simulink model "HAE"  (R2018a)
settings: Solver=ode4  StartTime=0  StopTime=2  MaxStep=1e-4  RelTol=1e-3
InitFcn:
  | close
  | clear
  | clc
  | Sc=128
  | f=60;
  | T=1/f;
  | Ts=1/(f*Sc);
  | Vr=6500
  | V_v=[1    0.4    1          0.6       1       0.6       1       0.75   0.95]
  | T_v=[0   20/f  70/f    200/f   300/f     330/f   400/f   500/f  10]
  | S_time=60/f*20.5
  | V_R=3;
  | Tf=3
  | T_lc=3
  | set_param('HAE/EMISOR-RECEPTOR/TCP_IP_RX1/ESCRITURA', 'Value','0')
  | set_param('HAE/EMISOR-RECEPTOR/TCP_IP_RX1/RETARDO', 'Value','0')
  | run script_client_1_inicio2.m
undefined symbols (not defined in the file or in its folder): D11, Delta, DiscIntNeverNeededParam, Int, Ip1
libraries: powerlib x68, simulink x12, powerlib_meascontrol x6, libreria_comunicaciones_cliente2 x2, libreria_medidores2 x1
(part 3 of 5)

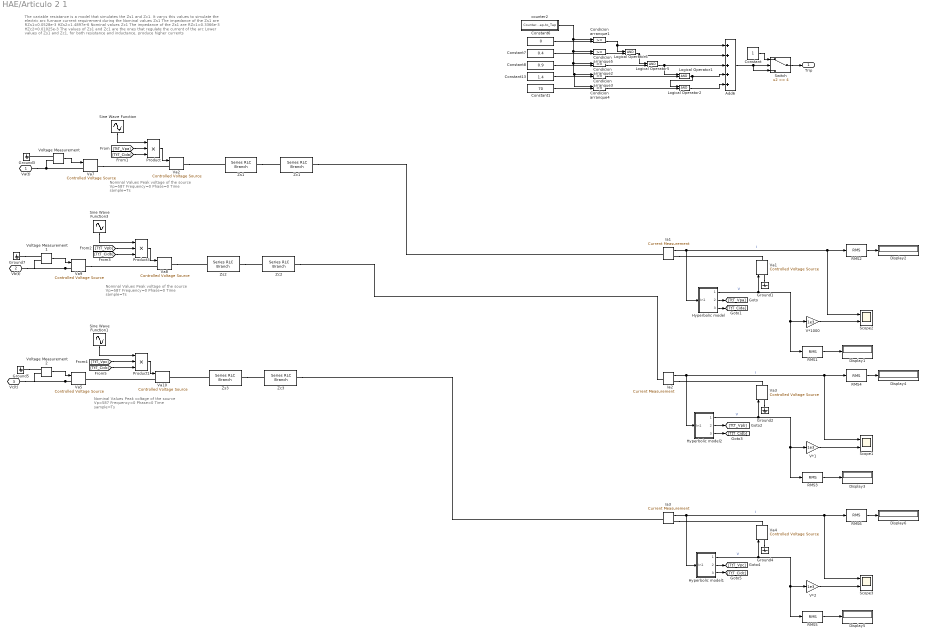
== system HAE/Articulo 2 1 ==
  note: The variable resistance is a model that simulates the Zs1 and Zc1. It varys this values to simulate the electric arc furnace current requirement during the
      |
      | Nominal values  Zs1
      | The impedance of the Zs1 are
      | RZs1=0.0528e-3
      | HZs2=1.4897e-6
      |
      | Nominal values Zc1
      | The impedance of the Zs1 are
      | RZc1=0.3366e-3
      | HZc2=0.01025e-3
      |
      |
      | The values of Zs1 and Zc1 are the ones that regulate the current of the arc
      |
      | Lower values of Zs1 and Zc1, for both resistance and inductance, produce higher currents
  note: Nominal Values
      |
      | Peak voltage of the source Vp=587
      | Frequency=0
      | Phase=0
      | Time sample=Ts
  note: Nominal Values
      |
      | Peak voltage of the source Vp=587
      | Frequency=0
      | Phase=0
      | Time sample=Ts
  note: Nominal Values
      |
      | Peak voltage of the source Vp=587
      | Frequency=0
      | Phase=0
      | Time sample=Ts
  Add6 : Sum  Inputs=+++++
  Condicion arranque{1..5} (5 alike) : RelationalOperator  OutDataTypeStr=boolean  RndMeth=Nearest
  Constant : Constant
  Constant1 : Constant  Value=70  VectorParams1D=off  SampleTime=Ts
  Constant13 : Constant  Value=1.4  VectorParams1D=off  SampleTime=Ts
  Constant6 : Constant  Value=0  VectorParams1D=off  SampleTime=Ts
  Constant7 : Constant  Value=0.4  VectorParams1D=off  SampleTime=Ts
  Constant8 : Constant  Value=0.9  VectorParams1D=off  SampleTime=Ts
  Display{1..6} (6 alike) : Display
  Ground{1..5,7} (6 alike) : powerlib/Elements/Ground  LConnTagsString=a
  Hyperbolic model : Subsystem
  Hyperbolic model1 : Subsystem
  Hyperbolic model2 : Subsystem
  Ia1 : powerlib/Measurements/Current Measurement  PhasorSimulation=off  OutputType=Complex  PSBequivalent=0
  Ia2 : powerlib/Measurements/Current Measurement  PhasorSimulation=off  OutputType=Complex  PSBequivalent=0
  Ia3 : powerlib/Measurements/Current Measurement  PhasorSimulation=off  OutputType=Complex  PSBequivalent=0
  Logical Operator{1..2,5..6} (4 alike) : Logic  AllPortsSameDT=off  OutDataTypeStr=boolean
  Product : Product  Inputs=3
  Product1 : Product  Inputs=3
  Product3 : Product  Inputs=3
  RMS{1..6} (6 alike) : powerlib_meascontrol/Measurements/RMS  TrueRMS=on  Freq=60  RMSInit=120  Ts=Ts
  Scope1 : Scope  NumInputPorts=2
  Scope2 : Scope  NumInputPorts=2
  Scope3 : Scope  NumInputPorts=2
  Sine Wave Function : Sin  Amplitude=Vp  Frequency=60*2*pi  Phase=pi/8  SampleTime=Ts
  Sine Wave Function1 : Sin  Amplitude=Vp  Frequency=60*2*pi  Phase=-2*pi/3  SampleTime=Ts
  Sine Wave Function3 : Sin  Amplitude=Vp  Frequency=60*2*pi  Phase=2*pi/3  SampleTime=Ts
  Switch : Switch  Threshold=4
  V*1 : Gain  Gain=1e3
  V*1000 : Gain  Gain=1e3
  V*2 : Gain  Gain=1e3
  Va1 : powerlib/Electrical Sources/Controlled Voltage Source  Initialize=on  Source_Type=AC  Amplitude=0  Phase=0  Frequency=0  Measurements=None
  Va{2,5,7..10} (6 alike) : powerlib/Electrical Sources/Controlled Voltage Source  Initialize=on  Source_Type=AC  Amplitude=570  Phase=0  Frequency=60  Measurements=None
  Va3 : powerlib/Electrical Sources/Controlled Voltage Source  Initialize=on  Source_Type=AC  Amplitude=0  Phase=0  Frequency=0  Measurements=None
  Va4 : powerlib/Electrical Sources/Controlled Voltage Source  Initialize=on  Source_Type=AC  Amplitude=0  Phase=0  Frequency=0  Measurements=None
  Voltage Measurement : powerlib/Measurements/Voltage Measurement  PhasorSimulation=off  OutputType=Complex  PSBequivalent=0
  Voltage Measurement1 : powerlib/Measurements/Voltage Measurement  PhasorSimulation=off  OutputType=Complex  PSBequivalent=0
  Voltage Measurement2 : powerlib/Measurements/Voltage Measurement  PhasorSimulation=off  OutputType=Complex  PSBequivalent=0
  Zc1 : powerlib/Elements/Series RLC Branch  LConnTagsString=__new0  RConnTagsString=__new0  BranchType=RL  Resistance=RZc1  Inductance=HZc1  SetiL0=off  InitialCurrent=0  Capacitance=0  Setx0=off  InitialVoltage=0  Measurements=None
  Zc2 : powerlib/Elements/Series RLC Branch  LConnTagsString=__new0  RConnTagsString=__new0  BranchType=RL  Resistance=RZc1  Inductance=HZc1  SetiL0=off  InitialCurrent=0  Capacitance=0  Setx0=off  InitialVoltage=0  Measurements=None
  Zc3 : powerlib/Elements/Series RLC Branch  LConnTagsString=__new0  RConnTagsString=__new0  BranchType=RL  Resistance=RZc1  Inductance=HZc1  SetiL0=off  InitialCurrent=0  Capacitance=0  Setx0=off  InitialVoltage=0  Measurements=None
  Zs1 : powerlib/Elements/Series RLC Branch  LConnTagsString=__new0  RConnTagsString=__new0  BranchType=RL  Resistance=RZs1  Inductance=HZs1  SetiL0=off  InitialCurrent=20e3  Capacitance=0  Setx0=off  InitialVoltage=0  Measurements=None
  Zs2 : powerlib/Elements/Series RLC Branch  LConnTagsString=__new0  RConnTagsString=__new0  BranchType=RL  Resistance=RZs1  Inductance=HZs1  SetiL0=off  InitialCurrent=20e3  Capacitance=0  Setx0=off  InitialVoltage=0  Measurements=None
  Zs3 : powerlib/Elements/Series RLC Branch  LConnTagsString=__new0  RConnTagsString=__new0  BranchType=RL  Resistance=RZs1  Inductance=HZs1  SetiL0=off  InitialCurrent=20e3  Capacitance=0  Setx0=off  InitialVoltage=0  Measurements=None
  counter2 : Subsystem
  Va(t) : PMIOPort  Side=Left
  Vb(t) : PMIOPort  Port=2  Side=Left
  Vc(t) : PMIOPort  Port=3  Side=Left
  Trip : Outport
  wires:
  [TtT_Cida] -> Product/3
  Hyperbolic model/3(TtT_Cid) -> [TtT_Cida]
  [TtT_Vpa] -> Product/2
  Hyperbolic model/2(TtT_Vp) -> [TtT_Vpa]
  Product/1 -> Va2/1
  Sine Wave Function/1 -> Product/1
  Ia1/1 -> RMS2/1, Scope2/1, Hyperbolic model/1(In1)  "I"
  RMS2/1 -> Display2/1
  RMS1/1 -> Display1/1
  V*1000/1 -> Scope2/2
  Hyperbolic model/1(Varc) -> V*1000/1, RMS1/1, Va1/1  "V"
  Hyperbolic model2/3(TtT_Cid) -> [TtT_Cidb]
  Hyperbolic model2/2(TtT_Vp) -> [TtT_Vpb]
  Ia2/1 -> Hyperbolic model2/1(In1), RMS4/1, Scope1/1  "I"
  RMS4/1 -> Display4/1
  RMS3/1 -> Display3/1
  V*1/1 -> Scope1/2
  Hyperbolic model2/1(Varc) -> V*1/1, RMS3/1, Va3/1  "V"
  Hyperbolic model1/3(TtT_Cid) -> [TtT_Cidc]
  Hyperbolic model1/2(TtT_Vp) -> [TtT_Vpc]
  Ia3/1 -> Hyperbolic model1/1(In1), RMS6/1, Scope3/1  "I"
  RMS6/1 -> Display6/1
  RMS5/1 -> Display5/1
  V*2/1 -> Scope3/2
  Hyperbolic model1/1(Varc) -> V*2/1, RMS5/1, Va4/1  "V"
  Voltage Measurement/1 -> Va7/1
  Product3/1 -> Va8/1
  Sine Wave Function3/1 -> Product3/1
  Voltage Measurement1/1 -> Va9/1
  [TtT_Vpb] -> Product3/2
  [TtT_Cidb] -> Product3/3
  Product1/1 -> Va10/1
  Sine Wave Function1/1 -> Product1/1
  Voltage Measurement2/1 -> Va5/1
  [TtT_Vpc] -> Product1/2
  [TtT_Cidc] -> Product1/3
  Add6/1 -> Switch/3, Switch/2
  Constant13/1 -> Condicion arranque3/2
  Condicion arranque1/1 -> Logical Operator6/1, Add6/1
  Condicion arranque3/1 -> Logical Operator1/2
  Logical Operator6/1 -> Add6/2, Logical Operator5/1
  Condicion arranque5/1 -> Logical Operator6/2
  Condicion arranque2/1 -> Logical Operator5/2
  Logical Operator5/1 -> Logical Operator1/1, Add6/3
  Constant6/1 -> Condicion arranque1/2
  Constant8/1 -> Condicion arranque2/2
  Constant7/1 -> Condicion arranque5/2
  Logical Operator1/1 -> Logical Operator2/1, Add6/4
  counter2/1(Counter Tap-to_Tap) -> Condicion arranque5/1, Condicion arranque4/1, Condicion arranque3/1, Condicion arranque2/1, Condicion arranque1/1
  Logical Operator2/1 -> Add6/5
  Condicion arranque4/1 -> Logical Operator2/2
  Constant1/1 -> Condicion arranque4/2
  Switch/1 -> Trip/1
  Constant/1 -> Switch/1
  connections:
  Zc3/RConn1 -- Ia3/LConn1
  Zc2/RConn1 -- Ia2/LConn1
  Zc1/RConn1 -- Ia1/LConn1
  Va1/LConn1 -- Ground1/LConn1
  Zs1/RConn1 -- Zc1/LConn1
  Ia1/RConn1 -- Va1/RConn1
  Va8/RConn1 -- Zs2/LConn1
  Va3/LConn1 -- Ground2/LConn1
  Zs2/RConn1 -- Zc2/LConn1
  Ia2/RConn1 -- Va3/RConn1
  Va4/LConn1 -- Ground4/LConn1
  Zs3/RConn1 -- Zc3/LConn1
  Ia3/RConn1 -- Va4/RConn1
  Va2/RConn1 -- Zs1/LConn1
  Va(t)/RConn1 -- Voltage Measurement/LConn2 -- Va7/LConn1
  Va7/RConn1 -- Va2/LConn1
  Voltage Measurement/LConn1 -- Ground3/LConn1
  Va9/LConn1 -- Vb(t)/RConn1 -- Voltage Measurement1/LConn2
  Va9/RConn1 -- Va8/LConn1
  Ground7/LConn1 -- Voltage Measurement1/LConn1
  Va5/LConn1 -- Vc(t)/RConn1 -- Voltage Measurement2/LConn2
  Ground5/LConn1 -- Voltage Measurement2/LConn1
  Va10/LConn1 -- Va5/RConn1
  Zs3/LConn1 -- Va10/RConn1

== system HAE/EMISOR-RECEPTOR ==
  note: Transmisión de datos
  note: Recepción de datos
  In1 : Inport
  Data Type Conversion : DataTypeConversion  OutDataTypeStr=double
  Scope3 : Scope
  TCP_IP_RX1 : libreria_comunicaciones_cliente2/TCP_IP_RX1  SystemSampleTime=-1
      link override ESCRITURA: Value=client_1.dato_lectura
      link override RETARDO: Value=e
  TCP_IP_TX1 : libreria_comunicaciones_cliente2/TCP_IP_TX1  SystemSampleTime=-1
  Out1 : Outport
  wires:
  TCP_IP_RX1/1 -> Out1/1
  Data Type Conversion/1 -> TCP_IP_TX1/1
  In1/1 -> Scope3/1, Data Type Conversion/1

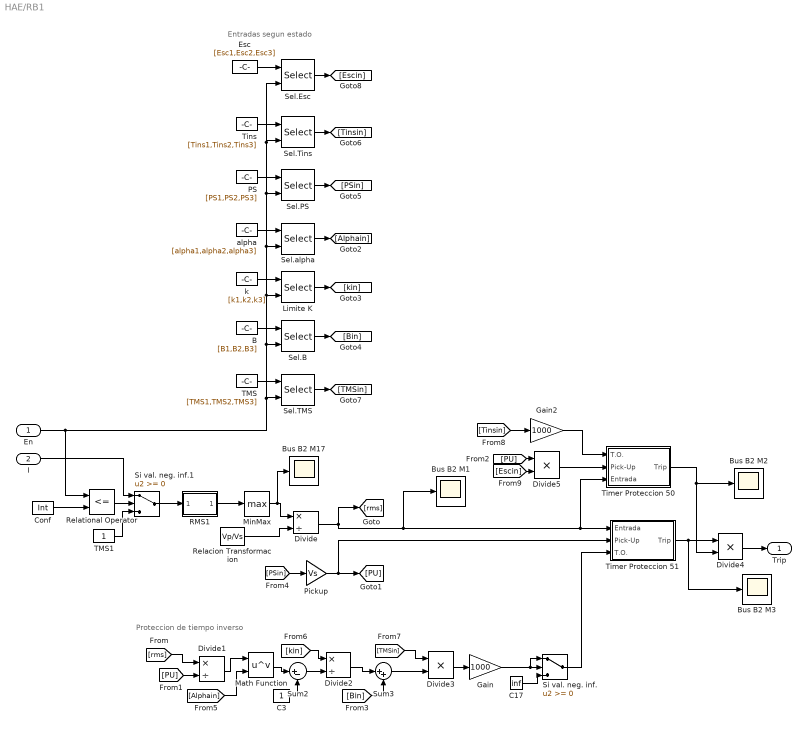
== system HAE/RB1 ==
  note: Proteccion de tiempo inverso
  note: Entradas segun estado
  En : Inport
  I : Inport  Port=2
  B : Constant  Value=[B1,B2,B3]
  Bus B2 M{1..3,17} (4 alike) : Scope
  C17 : Constant  Value=inf
  C3 : Constant
  Conf : Constant  Value=Int
  Divide : Product  Inputs=*/
  Divide1 : Product  Inputs=*/
  Divide2 : Product  Inputs=*/
  Divide3 : Product  Inputs=**
  Divide4 : Product  Inputs=**
  Divide5 : Product  Inputs=**
  Esc : Constant  Value=[Esc1,Esc2,Esc3]
  Gain : Gain  Gain=1000
  Gain2 : Gain  Gain=1000
  Limite K : Selector  InputPortWidth=3  IndexOptions=Index vector (port)  Indices=[1 2 3]  OutputSizes=1
  Math Function : Math  Operator=pow  SaturateOnIntegerOverflow=on
  MinMax : MinMax  Function=max
  PS : Constant  Value=[PS1,PS2,PS3]
  Pickup : Gain  Gain=Vs
  RMS1 : Subsystem
  Relacion Transformacion : Constant  Value=Vp/Vs
  Relational Operator : RelationalOperator  Operator=<=  OutDataTypeStr=boolean  RndMeth=Simplest
  Sel.B : Selector  InputPortWidth=3  IndexOptions=Index vector (port)  Indices=[1 2 3]  OutputSizes=1
  Sel.Esc : Selector  InputPortWidth=3  IndexOptions=Index vector (port)  Indices=[1 2 3]  OutputSizes=1
  Sel.PS : Selector  InputPortWidth=3  IndexOptions=Index vector (port)  Indices=[1 2 3]  OutputSizes=1
  Sel.TMS : Selector  InputPortWidth=3  IndexOptions=Index vector (port)  Indices=[1 2 3]  OutputSizes=1
  Sel.Tins : Selector  InputPortWidth=3  IndexOptions=Index vector (port)  Indices=[1 2 3]  OutputSizes=1
  Sel.alpha : Selector  InputPortWidth=3  IndexOptions=Index vector (port)  Indices=[1 2 3]  OutputSizes=1
  Si val. neg. inf. : Switch
  Si val. neg. inf.1 : Switch
  Sum2 : Sum  Inputs=|+-
  Sum3 : Sum  Inputs=|++
  TMS : Constant  Value=[TMS1,TMS2,TMS3]
  TMS1 : Constant
  Timer Proteccion 50 : Subsystem
  Timer Proteccion 51 : Subsystem
  Tins : Constant  Value=[Tins1,Tins2,Tins3]
  alpha : Constant  Value=[alpha1,alpha2,alpha3]
  k : Constant  Value=[k1,k2,k3]
  Trip : Outport
  wires:
  En/1 -> Relational Operator/1, Sel.TMS/2, Sel.B/2, Limite K/2, Sel.alpha/2, Sel.PS/2, Sel.Tins/2, Sel.Esc/2
  Divide4/1 -> Trip/1
  Tins/1 -> Sel.Tins/1
  [Escin] -> Divide5/2
  Sel.Esc/1 -> [Escin]
  C17/1 -> Si val. neg. inf./3
  Esc/1 -> Sel.Esc/1
  Math Function/1 -> Sum2/1
  [kin] -> Divide2/1
  Timer Proteccion 50/1(Trip) -> Bus B2 M2/1, Divide4/2
  [PSin] -> Pickup/1
  Si val. neg. inf./1 -> Timer Proteccion 51/3(T.O.)
  Sel.TMS/1 -> [TMSin]
  PS/1 -> Sel.PS/1
  [Tinsin] -> Gain2/1
  Timer Proteccion 51/1(Trip) -> Bus B2 M3/1, Divide4/1
  [Alphain] -> Math Function/2
  Divide3/1 -> Gain/1
  [PU] -> Divide1/2
  [PU] -> Divide5/1
  B/1 -> Sel.B/1
  Divide5/1 -> Timer Proteccion 50/2(Pick-Up)
  Divide2/1 -> Sum3/1
  Gain2/1 -> Timer Proteccion 50/1(T.O.)
  Gain/1 -> Si val. neg. inf./1, Si val. neg. inf./2
  Sum3/1 -> Divide3/2
  Sel.alpha/1 -> [Alphain]
  [Bin] -> Sum3/2
  Relacion Transformacion/1 -> Divide/2
  Divide/1 -> Bus B2 M1/1, Timer Proteccion 51/1(Entrada), Timer Proteccion 50/3(Entrada), [rms]
  Sum2/1 -> Divide2/2
  Divide1/1 -> Math Function/1
  Limite K/1 -> [kin]
  [rms] -> Divide1/1
  Pickup/1 -> Timer Proteccion 51/2(Pick-Up), [PU]
  Sel.B/1 -> [Bin]
  Sel.PS/1 -> [PSin]
  MinMax/1 -> Bus B2 M17/1, Divide/1
  RMS1/1(Out1) -> MinMax/1
  [TMSin] -> Divide3/1
  TMS/1 -> Sel.TMS/1
  C3/1 -> Sum2/2
  k/1 -> Limite K/1
  alpha/1 -> Sel.alpha/1
  Sel.Tins/1 -> [Tinsin]
  I/1 -> Si val. neg. inf.1/1
  Relational Operator/1 -> Si val. neg. inf.1/2
  Si val. neg. inf.1/1 -> RMS1/1(In1)
  Conf/1 -> Relational Operator/2
  TMS1/1 -> Si val. neg. inf.1/3

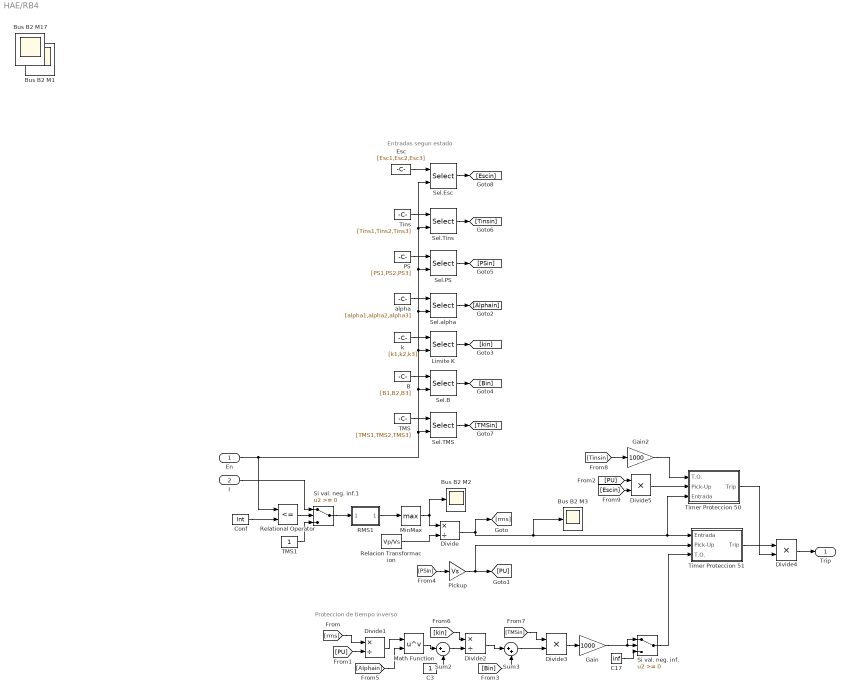
== system HAE/RB4 ==
  note: Entradas segun estado
  note: Proteccion de tiempo inverso
  En : Inport
  I : Inport  Port=2
  B : Constant  Value=[B1,B2,B3]
  Bus B2 M{1..3,17} (4 alike) : Scope
  C17 : Constant  Value=inf
  C3 : Constant
  Conf : Constant  Value=Int
  Divide : Product  Inputs=*/
  Divide1 : Product  Inputs=*/
  Divide2 : Product  Inputs=*/
  Divide3 : Product  Inputs=**
  Divide4 : Product  Inputs=**
  Divide5 : Product  Inputs=**
  Esc : Constant  Value=[Esc1,Esc2,Esc3]
  Gain : Gain  Gain=1000
  Gain2 : Gain  Gain=1000
  Limite K : Selector  InputPortWidth=3  IndexOptions=Index vector (port)  Indices=[1 2 3]  OutputSizes=1
  Math Function : Math  Operator=pow  SaturateOnIntegerOverflow=on
  MinMax : MinMax  Function=max
  PS : Constant  Value=[PS1,PS2,PS3]
  Pickup : Gain  Gain=Vs
  RMS1 : Subsystem
  Relacion Transformacion : Constant  Value=Vp/Vs
  Relational Operator : RelationalOperator  Operator=<=  OutDataTypeStr=boolean  RndMeth=Simplest
  Sel.B : Selector  InputPortWidth=3  IndexOptions=Index vector (port)  Indices=[1 2 3]  OutputSizes=1
  Sel.Esc : Selector  InputPortWidth=3  IndexOptions=Index vector (port)  Indices=[1 2 3]  OutputSizes=1
  Sel.PS : Selector  InputPortWidth=3  IndexOptions=Index vector (port)  Indices=[1 2 3]  OutputSizes=1
  Sel.TMS : Selector  InputPortWidth=3  IndexOptions=Index vector (port)  Indices=[1 2 3]  OutputSizes=1
  Sel.Tins : Selector  InputPortWidth=3  IndexOptions=Index vector (port)  Indices=[1 2 3]  OutputSizes=1
  Sel.alpha : Selector  InputPortWidth=3  IndexOptions=Index vector (port)  Indices=[1 2 3]  OutputSizes=1
  Si val. neg. inf. : Switch
  Si val. neg. inf.1 : Switch
  Sum2 : Sum  Inputs=|+-
  Sum3 : Sum  Inputs=|++
  TMS : Constant  Value=[TMS1,TMS2,TMS3]
  TMS1 : Constant
  Timer Proteccion 50 : Subsystem
  Timer Proteccion 51 : Subsystem
  Tins : Constant  Value=[Tins1,Tins2,Tins3]
  alpha : Constant  Value=[alpha1,alpha2,alpha3]
  k : Constant  Value=[k1,k2,k3]
  Trip : Outport
  wires:
  TMS1/1 -> Si val. neg. inf.1/3
  Conf/1 -> Relational Operator/2
  Si val. neg. inf.1/1 -> RMS1/1(In1)
  Relational Operator/1 -> Si val. neg. inf.1/2
  I/1 -> Si val. neg. inf.1/1
  Sel.Tins/1 -> [Tinsin]
  alpha/1 -> Sel.alpha/1
  k/1 -> Limite K/1
  C3/1 -> Sum2/2
  TMS/1 -> Sel.TMS/1
  [TMSin] -> Divide3/1
  RMS1/1(Out1) -> MinMax/1
  MinMax/1 -> Bus B2 M2/1, Divide/1
  Sel.PS/1 -> [PSin]
  Sel.B/1 -> [Bin]
  Pickup/1 -> [PU], Timer Proteccion 51/2(Pick-Up)
  [rms] -> Divide1/1
  Limite K/1 -> [kin]
  Divide1/1 -> Math Function/1
  Sum2/1 -> Divide2/2
  Divide/1 -> [rms], Bus B2 M3/1, Timer Proteccion 50/3(Entrada), Timer Proteccion 51/1(Entrada)
  Relacion Transformacion/1 -> Divide/2
  [Bin] -> Sum3/2
  Sel.alpha/1 -> [Alphain]
  Sum3/1 -> Divide3/2
  Gain/1 -> Si val. neg. inf./2, Si val. neg. inf./1
  Gain2/1 -> Timer Proteccion 50/1(T.O.)
  Divide2/1 -> Sum3/1
  Divide5/1 -> Timer Proteccion 50/2(Pick-Up)
  B/1 -> Sel.B/1
  [PU] -> Divide5/1
  [PU] -> Divide1/2
  Divide3/1 -> Gain/1
  [Alphain] -> Math Function/2
  Timer Proteccion 51/1(Trip) -> Divide4/1
  [Tinsin] -> Gain2/1
  PS/1 -> Sel.PS/1
  Sel.TMS/1 -> [TMSin]
  Si val. neg. inf./1 -> Timer Proteccion 51/3(T.O.)
  [PSin] -> Pickup/1
  Timer Proteccion 50/1(Trip) -> Divide4/2
  [kin] -> Divide2/1
  Math Function/1 -> Sum2/1
  Esc/1 -> Sel.Esc/1
  C17/1 -> Si val. neg. inf./3
  Sel.Esc/1 -> [Escin]
  [Escin] -> Divide5/2
  Tins/1 -> Sel.Tins/1
  Divide4/1 -> Trip/1
  En/1 -> Sel.Esc/2, Sel.Tins/2, Sel.PS/2, Sel.alpha/2, Limite K/2, Sel.B/2, Sel.TMS/2, Relational Operator/1

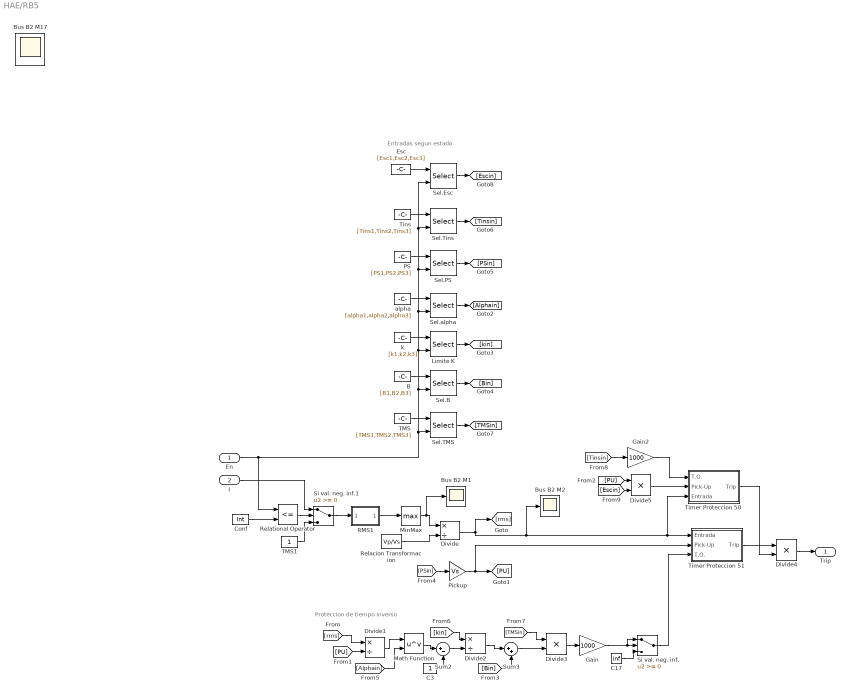
== system HAE/RB5 ==
  note: Proteccion de tiempo inverso
  note: Entradas segun estado
  En : Inport
  I : Inport  Port=2
  B : Constant  Value=[B1,B2,B3]
  Bus B2 M1 : Scope
  Bus B2 M17 : Scope
  Bus B2 M2 : Scope
  C17 : Constant  Value=inf
  C3 : Constant
  Conf : Constant  Value=Int
  Divide : Product  Inputs=*/
  Divide1 : Product  Inputs=*/
  Divide2 : Product  Inputs=*/
  Divide3 : Product  Inputs=**
  Divide4 : Product  Inputs=**
  Divide5 : Product  Inputs=**
  Esc : Constant  Value=[Esc1,Esc2,Esc3]
  Gain : Gain  Gain=1000
  Gain2 : Gain  Gain=1000
  Limite K : Selector  InputPortWidth=3  IndexOptions=Index vector (port)  Indices=[1 2 3]  OutputSizes=1
  Math Function : Math  Operator=pow  SaturateOnIntegerOverflow=on
  MinMax : MinMax  Function=max
  PS : Constant  Value=[PS1,PS2,PS3]
  Pickup : Gain  Gain=Vs
  RMS1 : Subsystem
  Relacion Transformacion : Constant  Value=Vp/Vs
  Relational Operator : RelationalOperator  Operator=<=  OutDataTypeStr=boolean  RndMeth=Simplest
  Sel.B : Selector  InputPortWidth=3  IndexOptions=Index vector (port)  Indices=[1 2 3]  OutputSizes=1
  Sel.Esc : Selector  InputPortWidth=3  IndexOptions=Index vector (port)  Indices=[1 2 3]  OutputSizes=1
  Sel.PS : Selector  InputPortWidth=3  IndexOptions=Index vector (port)  Indices=[1 2 3]  OutputSizes=1
  Sel.TMS : Selector  InputPortWidth=3  IndexOptions=Index vector (port)  Indices=[1 2 3]  OutputSizes=1
  Sel.Tins : Selector  InputPortWidth=3  IndexOptions=Index vector (port)  Indices=[1 2 3]  OutputSizes=1
  Sel.alpha : Selector  InputPortWidth=3  IndexOptions=Index vector (port)  Indices=[1 2 3]  OutputSizes=1
  Si val. neg. inf. : Switch
  Si val. neg. inf.1 : Switch
  Sum2 : Sum  Inputs=|+-
  Sum3 : Sum  Inputs=|++
  TMS : Constant  Value=[TMS1,TMS2,TMS3]
  TMS1 : Constant
  Timer Proteccion 50 : Subsystem
  Timer Proteccion 51 : Subsystem
  Tins : Constant  Value=[Tins1,Tins2,Tins3]
  alpha : Constant  Value=[alpha1,alpha2,alpha3]
  k : Constant  Value=[k1,k2,k3]
  Trip : Outport
  wires:
  En/1 -> Relational Operator/1, Sel.TMS/2, Sel.B/2, Limite K/2, Sel.alpha/2, Sel.PS/2, Sel.Tins/2, Sel.Esc/2
  Divide4/1 -> Trip/1
  Tins/1 -> Sel.Tins/1
  [Escin] -> Divide5/2
  Sel.Esc/1 -> [Escin]
  C17/1 -> Si val. neg. inf./3
  Esc/1 -> Sel.Esc/1
  Math Function/1 -> Sum2/1
  [kin] -> Divide2/1
  Timer Proteccion 50/1(Trip) -> Divide4/2
  [PSin] -> Pickup/1
  Si val. neg. inf./1 -> Timer Proteccion 51/3(T.O.)
  Sel.TMS/1 -> [TMSin]
  PS/1 -> Sel.PS/1
  [Tinsin] -> Gain2/1
  Timer Proteccion 51/1(Trip) -> Divide4/1
  [Alphain] -> Math Function/2
  Divide3/1 -> Gain/1
  [PU] -> Divide1/2
  [PU] -> Divide5/1
  B/1 -> Sel.B/1
  Divide5/1 -> Timer Proteccion 50/2(Pick-Up)
  Divide2/1 -> Sum3/1
  Gain2/1 -> Timer Proteccion 50/1(T.O.)
  Gain/1 -> Si val. neg. inf./1, Si val. neg. inf./2
  Sum3/1 -> Divide3/2
  Sel.alpha/1 -> [Alphain]
  [Bin] -> Sum3/2
  Relacion Transformacion/1 -> Divide/2
  Divide/1 -> Bus B2 M2/1, Timer Proteccion 51/1(Entrada), Timer Proteccion 50/3(Entrada), [rms]
  Sum2/1 -> Divide2/2
  Divide1/1 -> Math Function/1
  Limite K/1 -> [kin]
  [rms] -> Divide1/1
  Pickup/1 -> Timer Proteccion 51/2(Pick-Up), [PU]
  Sel.B/1 -> [Bin]
  Sel.PS/1 -> [PSin]
  MinMax/1 -> Bus B2 M1/1, Divide/1
  RMS1/1(Out1) -> MinMax/1
  [TMSin] -> Divide3/1
  TMS/1 -> Sel.TMS/1
  C3/1 -> Sum2/2
  k/1 -> Limite K/1
  alpha/1 -> Sel.alpha/1
  Sel.Tins/1 -> [Tinsin]
  I/1 -> Si val. neg. inf.1/1
  Relational Operator/1 -> Si val. neg. inf.1/2
  Si val. neg. inf.1/1 -> RMS1/1(In1)
  Conf/1 -> Relational Operator/2
  TMS1/1 -> Si val. neg. inf.1/3

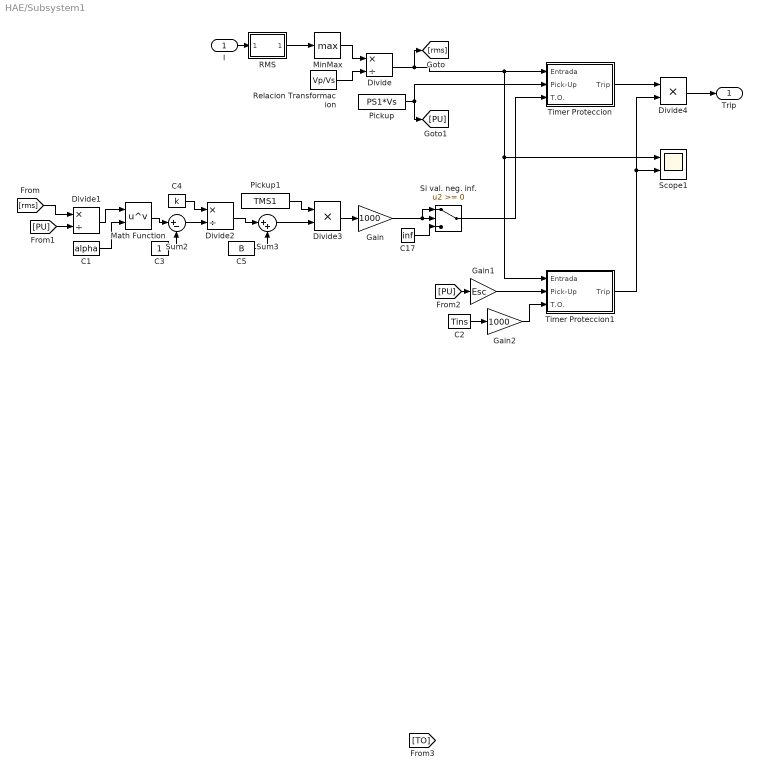
== system HAE/Subsystem1 ==
  I : Inport
  C1 : Constant  Value=alpha
  C17 : Constant  Value=inf
  C2 : Constant  Value=Tins
  C3 : Constant
  C4 : Constant  Value=k
  C5 : Constant  Value=B
  Divide : Product  Inputs=*/
  Divide1 : Product  Inputs=*/
  Divide2 : Product  Inputs=*/
  Divide3 : Product  Inputs=**
  Divide4 : Product  Inputs=**
  Gain : Gain  Gain=1000
  Gain1 : Gain  Gain=Esc
  Gain2 : Gain  Gain=1000
  Math Function : Math  Operator=pow  SaturateOnIntegerOverflow=on
  MinMax : MinMax  Function=max
  Pickup : Constant  Value=PS1*Vs
  Pickup1 : Constant  Value=TMS1
  RMS : Subsystem
  Relacion Transformacion : Constant  Value=Vp/Vs
  Scope1 : Scope  NumInputPorts=2
  Si val. neg. inf. : Switch
  Sum2 : Sum  Inputs=|+-
  Sum3 : Sum  Inputs=|++
  Timer Proteccion : Subsystem
  Timer Proteccion1 : Subsystem
  Trip : Outport
  wires:
  [PU] -> Divide1/2
  C1/1 -> Math Function/2
  C3/1 -> Sum2/2
  Pickup1/1 -> Divide3/1
  Divide2/1 -> Sum3/1
  Sum2/1 -> Divide2/2
  Math Function/1 -> Sum2/1
  C5/1 -> Sum3/2
  Pickup/1 -> Timer Proteccion/2(Pick-Up), [PU]
  Relacion Transformacion/1 -> Divide/2
  C4/1 -> Divide2/1
  Divide1/1 -> Math Function/1
  Sum3/1 -> Divide3/2
  Divide/1 -> Scope1/1, Timer Proteccion1/1(Entrada), Timer Proteccion/1(Entrada), [rms]
  [rms] -> Divide1/1
  I/1 -> RMS/1(In1)
  MinMax/1 -> Divide/1
  Divide3/1 -> Gain/1
  Gain/1 -> Si val. neg. inf./1, Si val. neg. inf./2
  RMS/1(Out1) -> MinMax/1
  C17/1 -> Si val. neg. inf./3
  Si val. neg. inf./1 -> Timer Proteccion/3(T.O.)
  [PU] -> Gain1/1
  Gain1/1 -> Timer Proteccion1/2(Pick-Up)
  Divide4/1 -> Trip/1
  Timer Proteccion/1(Trip) -> Divide4/1
  Timer Proteccion1/1(Trip) -> Scope1/2, Divide4/2
  C2/1 -> Gain2/1
  Gain2/1 -> Timer Proteccion1/3(T.O.)

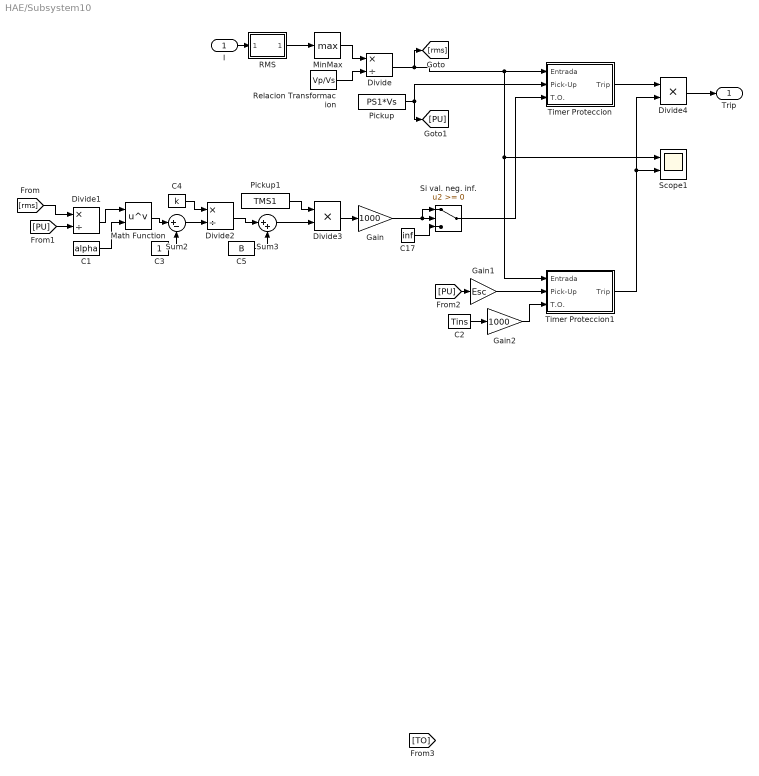
== system HAE/Subsystem10 ==
  I : Inport
  C1 : Constant  Value=alpha
  C17 : Constant  Value=inf
  C2 : Constant  Value=Tins
  C3 : Constant
  C4 : Constant  Value=k
  C5 : Constant  Value=B
  Divide : Product  Inputs=*/
  Divide1 : Product  Inputs=*/
  Divide2 : Product  Inputs=*/
  Divide3 : Product  Inputs=**
  Divide4 : Product  Inputs=**
  Gain : Gain  Gain=1000
  Gain1 : Gain  Gain=Esc
  Gain2 : Gain  Gain=1000
  Math Function : Math  Operator=pow  SaturateOnIntegerOverflow=on
  MinMax : MinMax  Function=max
  Pickup : Constant  Value=PS1*Vs
  Pickup1 : Constant  Value=TMS1
  RMS : Subsystem
  Relacion Transformacion : Constant  Value=Vp/Vs
  Scope1 : Scope  NumInputPorts=2
  Si val. neg. inf. : Switch
  Sum2 : Sum  Inputs=|+-
  Sum3 : Sum  Inputs=|++
  Timer Proteccion : Subsystem
  Timer Proteccion1 : Subsystem
  Trip : Outport
  wires:
  [PU] -> Divide1/2
  C1/1 -> Math Function/2
  C3/1 -> Sum2/2
  Pickup1/1 -> Divide3/1
  Divide2/1 -> Sum3/1
  Sum2/1 -> Divide2/2
  Math Function/1 -> Sum2/1
  C5/1 -> Sum3/2
  Pickup/1 -> Timer Proteccion/2(Pick-Up), [PU]
  Relacion Transformacion/1 -> Divide/2
  C4/1 -> Divide2/1
  Divide1/1 -> Math Function/1
  Sum3/1 -> Divide3/2
  Divide/1 -> Scope1/1, Timer Proteccion1/1(Entrada), Timer Proteccion/1(Entrada), [rms]
  [rms] -> Divide1/1
  I/1 -> RMS/1(In1)
  MinMax/1 -> Divide/1
  Divide3/1 -> Gain/1
  Gain/1 -> Si val. neg. inf./1, Si val. neg. inf./2
  RMS/1(Out1) -> MinMax/1
  C17/1 -> Si val. neg. inf./3
  Si val. neg. inf./1 -> Timer Proteccion/3(T.O.)
  [PU] -> Gain1/1
  Gain1/1 -> Timer Proteccion1/2(Pick-Up)
  Divide4/1 -> Trip/1
  Timer Proteccion/1(Trip) -> Divide4/1
  Timer Proteccion1/1(Trip) -> Scope1/2, Divide4/2
  C2/1 -> Gain2/1
  Gain2/1 -> Timer Proteccion1/3(T.O.)

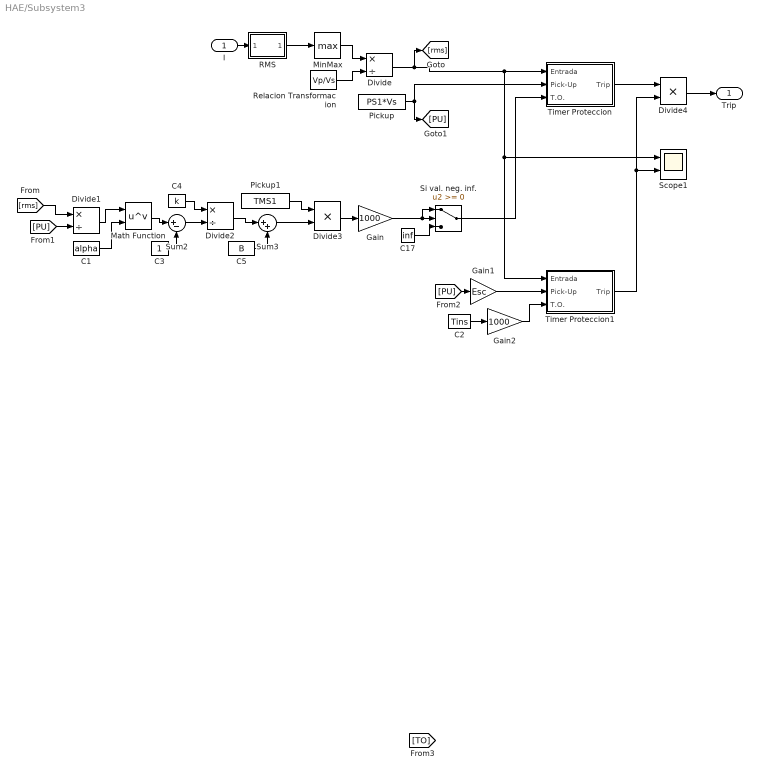
== system HAE/Subsystem3 ==
  I : Inport
  C1 : Constant  Value=alpha
  C17 : Constant  Value=inf
  C2 : Constant  Value=Tins
  C3 : Constant
  C4 : Constant  Value=k
  C5 : Constant  Value=B
  Divide : Product  Inputs=*/
  Divide1 : Product  Inputs=*/
  Divide2 : Product  Inputs=*/
  Divide3 : Product  Inputs=**
  Divide4 : Product  Inputs=**
  Gain : Gain  Gain=1000
  Gain1 : Gain  Gain=Esc
  Gain2 : Gain  Gain=1000
  Math Function : Math  Operator=pow  SaturateOnIntegerOverflow=on
  MinMax : MinMax  Function=max
  Pickup : Constant  Value=PS1*Vs
  Pickup1 : Constant  Value=TMS1
  RMS : Subsystem
  Relacion Transformacion : Constant  Value=Vp/Vs
  Scope1 : Scope  NumInputPorts=2
  Si val. neg. inf. : Switch
  Sum2 : Sum  Inputs=|+-
  Sum3 : Sum  Inputs=|++
  Timer Proteccion : Subsystem
  Timer Proteccion1 : Subsystem
  Trip : Outport
  wires:
  [PU] -> Divide1/2
  C1/1 -> Math Function/2
  C3/1 -> Sum2/2
  Pickup1/1 -> Divide3/1
  Divide2/1 -> Sum3/1
  Sum2/1 -> Divide2/2
  Math Function/1 -> Sum2/1
  C5/1 -> Sum3/2
  Pickup/1 -> Timer Proteccion/2(Pick-Up), [PU]
  Relacion Transformacion/1 -> Divide/2
  C4/1 -> Divide2/1
  Divide1/1 -> Math Function/1
  Sum3/1 -> Divide3/2
  Divide/1 -> Scope1/1, Timer Proteccion1/1(Entrada), Timer Proteccion/1(Entrada), [rms]
  [rms] -> Divide1/1
  I/1 -> RMS/1(In1)
  MinMax/1 -> Divide/1
  Divide3/1 -> Gain/1
  Gain/1 -> Si val. neg. inf./1, Si val. neg. inf./2
  RMS/1(Out1) -> MinMax/1
  C17/1 -> Si val. neg. inf./3
  Si val. neg. inf./1 -> Timer Proteccion/3(T.O.)
  [PU] -> Gain1/1
  Gain1/1 -> Timer Proteccion1/2(Pick-Up)
  Divide4/1 -> Trip/1
  Timer Proteccion/1(Trip) -> Divide4/1
  Timer Proteccion1/1(Trip) -> Scope1/2, Divide4/2
  C2/1 -> Gain2/1
  Gain2/1 -> Timer Proteccion1/3(T.O.)

== system HAE/Subsystem4 ==
  220/115 kV 67 MVA : powerlib/Elements/Three-Phase Transformer (Two Windings)  Winding1Connection=Delta (D11)  Winding2Connection=Yg  CoreType=Three single-phase transformers  SetSaturation=off  Hysteresis=off  DataFile='basic_model'  SetInitialFlux=off  Measurements=None  UNITS=pu  NominalPower=[67e6 60 ]  Winding1=[2.2e+05 0.00033931 0.010485]  Winding2=[115e+3 0.0057021 0.17621]  Rm=74.757  Lm=74.756  L0=0.5  Saturation=[0 0;0.01413 0.50702;2.8261 0.59153]  InitialFluxes=[0.33801 -0.33801 0.29576]  MoreParameters=off  BreakLoop=off  DataType=off  TransfoNumber=0
  Red 220 kV : powerlib/Measurements/Three-Phase V-I Measurement  VoltageMeasurement=phase-to-ground  SetLabelV=on  LabelV=V_TP  Vpu=off  VpuLL=off  CurrentMeasurement=yes  SetLabelI=on  LabelI=I_TP  Ipu=off  Pbase=100e6  Vbase=120e3  OutputType=Complex  PhasorSimulation=off  PSBequivalent=0
  TS 115 kV : powerlib/Measurements/Three-Phase V-I Measurement  VoltageMeasurement=phase-to-ground  SetLabelV=on  LabelV=V_TS  Vpu=off  VpuLL=off  CurrentMeasurement=yes  SetLabelI=on  LabelI=I_TS  Ipu=off  Pbase=100e6  Vbase=500e3  OutputType=Complex  PhasorSimulation=off  PSBequivalent=0
  Three-Phase PI Section Line1 : powerlib/Elements/Three-Phase PI Section Line  LConnTagsString=a|b|c  RConnTagsString=A|B|C  Frequency=60  Resistances=[0.2494 0.6766]  Inductances="[0.72521e-3  2.2365572e-3]"  Capacitances=[12.74e-9 7.751e-9]  Length=0.5
      settings: SourceProductName=Simscape Power Systems
  Three-Phase Source : powerlib/Electrical Sources/Three-Phase Source  InternalConnection=Yg  VoltagePhases=off  Voltage=220e3  PhaseAngle=0  Voltage_phases=[161e3 161e3 161e3]/sqrt(3)  PhaseAngles_phases=[0 -120 +120]  Frequency=60  NonIdealSource=on  SpecifyImpedance=on  Resistance=0.8929  Inductance=16.58e-3  ShortCircuitLevel=600e6  BaseVoltage=220e3  XRratio=10  BusType=swing  Pref=0  Qref=0  Prefabc=[10e3, 10e3, 10e3]  Qrefabc=[0, 0, 0]  Qmin=-inf  Qmax=inf
  Conn1 : PMIOPort  Side=Right
  Conn2 : PMIOPort  Port=2  Side=Right
  Conn3 : PMIOPort  Port=3  Side=Right
  connections:
  TS 115 kV/RConn3 -- Three-Phase PI Section Line1/LConn3
  Three-Phase Source/RConn3 -- Red 220 kV/LConn3
  220/115 kV 67 MVA/RConn1 -- TS 115 kV/LConn1
  Red 220 kV/RConn1 -- 220/115 kV 67 MVA/LConn1
  Three-Phase PI Section Line1/RConn3 -- Conn3/RConn1
  220/115 kV 67 MVA/RConn2 -- TS 115 kV/LConn2
  Three-Phase Source/RConn1 -- Red 220 kV/LConn1
  Red 220 kV/RConn2 -- 220/115 kV 67 MVA/LConn2
  220/115 kV 67 MVA/RConn3 -- TS 115 kV/LConn3
  Red 220 kV/LConn2 -- Three-Phase Source/RConn2
  TS 115 kV/RConn2 -- Three-Phase PI Section Line1/LConn2
  Red 220 kV/RConn3 -- 220/115 kV 67 MVA/LConn3
  TS 115 kV/RConn1 -- Three-Phase PI Section Line1/LConn1
  Three-Phase PI Section Line1/RConn2 -- Conn2/RConn1
  Three-Phase PI Section Line1/RConn1 -- Conn1/RConn1

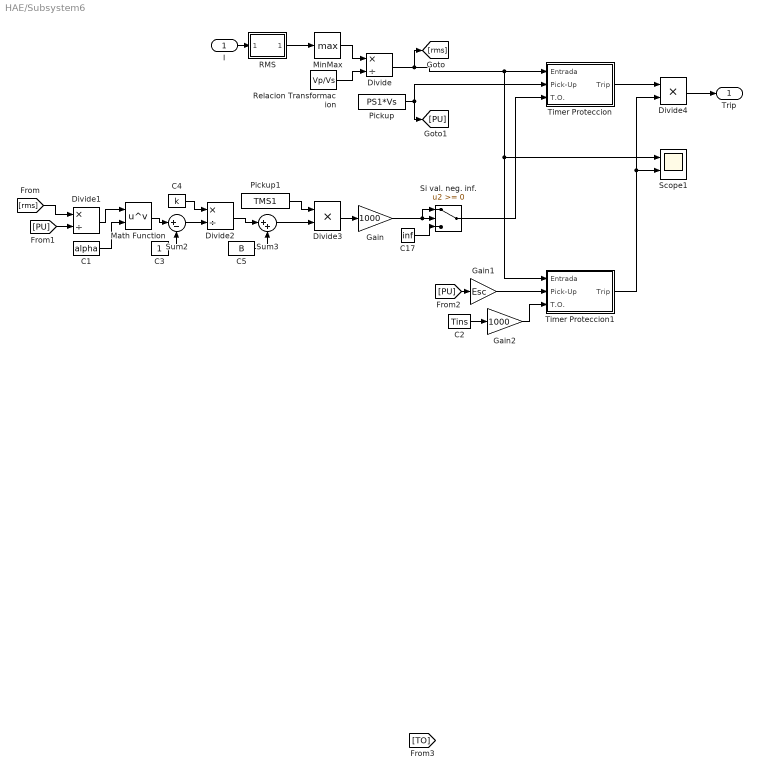
== system HAE/Subsystem6 ==
  I : Inport
  C1 : Constant  Value=alpha
  C17 : Constant  Value=inf
  C2 : Constant  Value=Tins
  C3 : Constant
  C4 : Constant  Value=k
  C5 : Constant  Value=B
  Divide : Product  Inputs=*/
  Divide1 : Product  Inputs=*/
  Divide2 : Product  Inputs=*/
  Divide3 : Product  Inputs=**
  Divide4 : Product  Inputs=**
  Gain : Gain  Gain=1000
  Gain1 : Gain  Gain=Esc
  Gain2 : Gain  Gain=1000
  Math Function : Math  Operator=pow  SaturateOnIntegerOverflow=on
  MinMax : MinMax  Function=max
  Pickup : Constant  Value=PS1*Vs
  Pickup1 : Constant  Value=TMS1
  RMS : Subsystem
  Relacion Transformacion : Constant  Value=Vp/Vs
  Scope1 : Scope  NumInputPorts=2
  Si val. neg. inf. : Switch
  Sum2 : Sum  Inputs=|+-
  Sum3 : Sum  Inputs=|++
  Timer Proteccion : Subsystem
  Timer Proteccion1 : Subsystem
  Trip : Outport
  wires:
  [PU] -> Divide1/2
  C1/1 -> Math Function/2
  C3/1 -> Sum2/2
  Pickup1/1 -> Divide3/1
  Divide2/1 -> Sum3/1
  Sum2/1 -> Divide2/2
  Math Function/1 -> Sum2/1
  C5/1 -> Sum3/2
  Pickup/1 -> Timer Proteccion/2(Pick-Up), [PU]
  Relacion Transformacion/1 -> Divide/2
  C4/1 -> Divide2/1
  Divide1/1 -> Math Function/1
  Sum3/1 -> Divide3/2
  Divide/1 -> Scope1/1, Timer Proteccion1/1(Entrada), Timer Proteccion/1(Entrada), [rms]
  [rms] -> Divide1/1
  I/1 -> RMS/1(In1)
  MinMax/1 -> Divide/1
  Divide3/1 -> Gain/1
  Gain/1 -> Si val. neg. inf./1, Si val. neg. inf./2
  RMS/1(Out1) -> MinMax/1
  C17/1 -> Si val. neg. inf./3
  Si val. neg. inf./1 -> Timer Proteccion/3(T.O.)
  [PU] -> Gain1/1
  Gain1/1 -> Timer Proteccion1/2(Pick-Up)
  Divide4/1 -> Trip/1
  Timer Proteccion/1(Trip) -> Divide4/1
  Timer Proteccion1/1(Trip) -> Scope1/2, Divide4/2
  C2/1 -> Gain2/1
  Gain2/1 -> Timer Proteccion1/3(T.O.)

== system HAE/Subsystem7 ==
  I : Inport
  C1 : Constant  Value=alpha
  C17 : Constant  Value=inf
  C2 : Constant  Value=Tins
  C3 : Constant
  C4 : Constant  Value=k
  C5 : Constant  Value=B
  Divide : Product  Inputs=*/
  Divide1 : Product  Inputs=*/
  Divide2 : Product  Inputs=*/
  Divide3 : Product  Inputs=**
  Divide4 : Product  Inputs=**
  Gain : Gain  Gain=1000
  Gain1 : Gain  Gain=Esc
  Gain2 : Gain  Gain=1000
  Math Function : Math  Operator=pow  SaturateOnIntegerOverflow=on
  MinMax : MinMax  Function=max
  Pickup : Constant  Value=PS1*Vs
  Pickup1 : Constant  Value=TMS1
  RMS : Subsystem
  Relacion Transformacion : Constant  Value=Vp/Vs
  Scope1 : Scope  NumInputPorts=2
  Si val. neg. inf. : Switch
  Sum2 : Sum  Inputs=|+-
  Sum3 : Sum  Inputs=|++
  Timer Proteccion : Subsystem
  Timer Proteccion1 : Subsystem
  Trip : Outport
  wires:
  [PU] -> Divide1/2
  C1/1 -> Math Function/2
  C3/1 -> Sum2/2
  Pickup1/1 -> Divide3/1
  Divide2/1 -> Sum3/1
  Sum2/1 -> Divide2/2
  Math Function/1 -> Sum2/1
  C5/1 -> Sum3/2
  Pickup/1 -> Timer Proteccion/2(Pick-Up), [PU]
  Relacion Transformacion/1 -> Divide/2
  C4/1 -> Divide2/1
  Divide1/1 -> Math Function/1
  Sum3/1 -> Divide3/2
  Divide/1 -> Scope1/1, Timer Proteccion1/1(Entrada), Timer Proteccion/1(Entrada), [rms]
  [rms] -> Divide1/1
  I/1 -> RMS/1(In1)
  MinMax/1 -> Divide/1
  Divide3/1 -> Gain/1
  Gain/1 -> Si val. neg. inf./1, Si val. neg. inf./2
  RMS/1(Out1) -> MinMax/1
  C17/1 -> Si val. neg. inf./3
  Si val. neg. inf./1 -> Timer Proteccion/3(T.O.)
  [PU] -> Gain1/1
  Gain1/1 -> Timer Proteccion1/2(Pick-Up)
  Divide4/1 -> Trip/1
  Timer Proteccion/1(Trip) -> Divide4/1
  Timer Proteccion1/1(Trip) -> Scope1/2, Divide4/2
  C2/1 -> Gain2/1
  Gain2/1 -> Timer Proteccion1/3(T.O.)

== system HAE/Subsystem8 ==
  I : Inport
  C1 : Constant  Value=alpha
  C17 : Constant  Value=inf
  C2 : Constant  Value=Tins
  C3 : Constant
  C4 : Constant  Value=k
  C5 : Constant  Value=B
  Divide : Product  Inputs=*/
  Divide1 : Product  Inputs=*/
  Divide2 : Product  Inputs=*/
  Divide3 : Product  Inputs=**
  Divide4 : Product  Inputs=**
  Gain : Gain  Gain=1000
  Gain1 : Gain  Gain=Esc
  Gain2 : Gain  Gain=1000
  Math Function : Math  Operator=pow  SaturateOnIntegerOverflow=on
  MinMax : MinMax  Function=max
  Pickup : Constant  Value=PS1*Vs
  Pickup1 : Constant  Value=TMS1
  RMS : Subsystem
  Relacion Transformacion : Constant  Value=Vp/Vs
  Scope1 : Scope  NumInputPorts=2
  Si val. neg. inf. : Switch
  Sum2 : Sum  Inputs=|+-
  Sum3 : Sum  Inputs=|++
  Timer Proteccion : Subsystem
  Timer Proteccion1 : Subsystem
  Trip : Outport
  wires:
  [PU] -> Divide1/2
  C1/1 -> Math Function/2
  C3/1 -> Sum2/2
  Pickup1/1 -> Divide3/1
  Divide2/1 -> Sum3/1
  Sum2/1 -> Divide2/2
  Math Function/1 -> Sum2/1
  C5/1 -> Sum3/2
  Pickup/1 -> Timer Proteccion/2(Pick-Up), [PU]
  Relacion Transformacion/1 -> Divide/2
  C4/1 -> Divide2/1
  Divide1/1 -> Math Function/1
  Sum3/1 -> Divide3/2
  Divide/1 -> Scope1/1, Timer Proteccion1/1(Entrada), Timer Proteccion/1(Entrada), [rms]
  [rms] -> Divide1/1
  I/1 -> RMS/1(In1)
  MinMax/1 -> Divide/1
  Divide3/1 -> Gain/1
  Gain/1 -> Si val. neg. inf./1, Si val. neg. inf./2
  RMS/1(Out1) -> MinMax/1
  C17/1 -> Si val. neg. inf./3
  Si val. neg. inf./1 -> Timer Proteccion/3(T.O.)
  [PU] -> Gain1/1
  Gain1/1 -> Timer Proteccion1/2(Pick-Up)
  Divide4/1 -> Trip/1
  Timer Proteccion/1(Trip) -> Divide4/1
  Timer Proteccion1/1(Trip) -> Scope1/2, Divide4/2
  C2/1 -> Gain2/1
  Gain2/1 -> Timer Proteccion1/3(T.O.)

== system HAE/Subsystem9 ==
  I : Inport
  C1 : Constant  Value=alpha
  C17 : Constant  Value=inf
  C2 : Constant  Value=Tins
  C3 : Constant
  C4 : Constant  Value=k
  C5 : Constant  Value=B
  Divide : Product  Inputs=*/
  Divide1 : Product  Inputs=*/
  Divide2 : Product  Inputs=*/
  Divide3 : Product  Inputs=**
  Divide4 : Product  Inputs=**
  Gain : Gain  Gain=1000
  Gain1 : Gain  Gain=Esc
  Gain2 : Gain  Gain=1000
  Math Function : Math  Operator=pow  SaturateOnIntegerOverflow=on
  MinMax : MinMax  Function=max
  Pickup : Constant  Value=PS1*Vs
  Pickup1 : Constant  Value=TMS1
  RMS : Subsystem
  Relacion Transformacion : Constant  Value=Vp/Vs
  Scope1 : Scope  NumInputPorts=2
  Si val. neg. inf. : Switch
  Sum2 : Sum  Inputs=|+-
  Sum3 : Sum  Inputs=|++
  Timer Proteccion : Subsystem
  Timer Proteccion1 : Subsystem
  Trip : Outport
  wires:
  [PU] -> Divide1/2
  C1/1 -> Math Function/2
  C3/1 -> Sum2/2
  Pickup1/1 -> Divide3/1
  Divide2/1 -> Sum3/1
  Sum2/1 -> Divide2/2
  Math Function/1 -> Sum2/1
  C5/1 -> Sum3/2
  Pickup/1 -> Timer Proteccion/2(Pick-Up), [PU]
  Relacion Transformacion/1 -> Divide/2
  C4/1 -> Divide2/1
  Divide1/1 -> Math Function/1
  Sum3/1 -> Divide3/2
  Divide/1 -> Scope1/1, Timer Proteccion1/1(Entrada), Timer Proteccion/1(Entrada), [rms]
  [rms] -> Divide1/1
  I/1 -> RMS/1(In1)
  MinMax/1 -> Divide/1
  Divide3/1 -> Gain/1
  Gain/1 -> Si val. neg. inf./1, Si val. neg. inf./2
  RMS/1(Out1) -> MinMax/1
  C17/1 -> Si val. neg. inf./3
  Si val. neg. inf./1 -> Timer Proteccion/3(T.O.)
  [PU] -> Gain1/1
  Gain1/1 -> Timer Proteccion1/2(Pick-Up)
  Divide4/1 -> Trip/1
  Timer Proteccion/1(Trip) -> Divide4/1
  Timer Proteccion1/1(Trip) -> Scope1/2, Divide4/2
  C2/1 -> Gain2/1
  Gain2/1 -> Timer Proteccion1/3(T.O.)

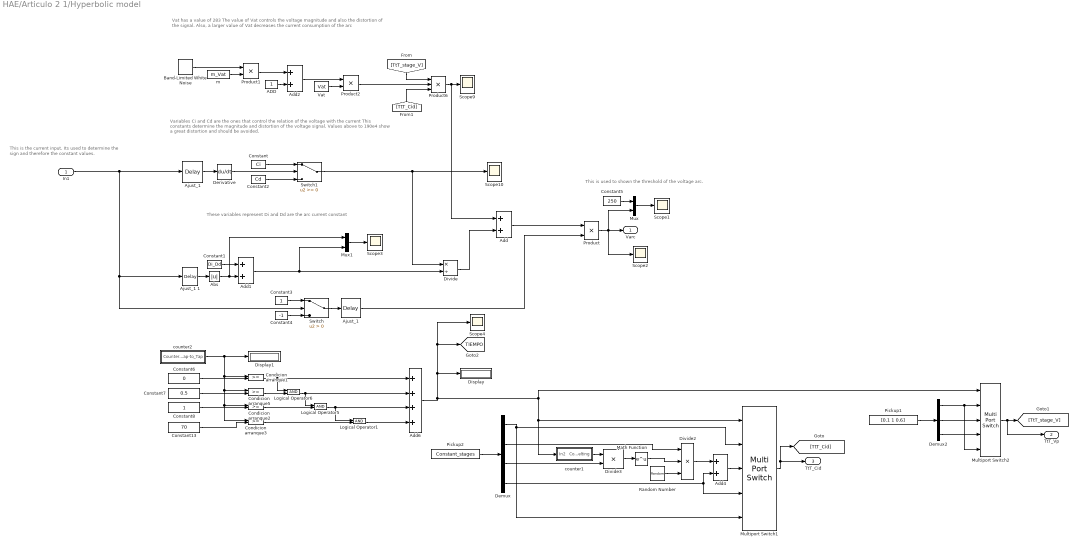
== system HAE/Articulo 2 1/Hyperbolic model ==
  note: Vat has a value of 283
      | The value of Vat controls the voltage magnitude and also the distortion of the signal.
      |
      | Also, a larger value of Vat decreases the current consumption of the arc
  note: Variables  Ci and Cd are the ones that control the relation of the voltage with the current
      |
      | This constants determine the magnitude and distortion of the voltage signal.
      |
      | Values above to 190e4 show a great distortion and should be avoided.
  note: These variables represent Di and Dd are the arc current constant
  note: This is used to shown the threshold of the voltage arc.
  note: This is the current input. Its used to determine the sign and therefore the constant values.
  In1 : Inport
  ADD : Constant  SampleTime=Ts
  Abs : Abs
  Add{,1..2,4} (4 alike) : Sum
  Add6 : Sum  Inputs=++++
  Ajust_1 : TransportDelay  DelayTime=1/(1024*60)
  "Ajust_1 " : TransportDelay  DelayTime=1/(1024*60)
  Ajust_1 1 : TransportDelay  DelayTime=1/(1024*60)
  Band-Limited White Noise : simulink/Sources/Band-Limited White Noise  Cov=[0.00005]  Ts=Ts  seed=[500]
  Condicion arranque{1..3,5} (4 alike) : RelationalOperator  OutDataTypeStr=boolean  RndMeth=Nearest
  Constant : Constant  Value=Ci  SampleTime=Ts
  Constant1 : Constant  Value=Di_Dd  SampleTime=Ts
  Constant13 : Constant  Value=70  VectorParams1D=off  SampleTime=Ts
  Constant2 : Constant  Value=Cd
  Constant3 : Constant
  Constant4 : Constant  Value=-1
  Constant5 : Constant  Value=250
  Constant6 : Constant  Value=0  VectorParams1D=off  SampleTime=Ts
  Constant7 : Constant  Value=0.5  VectorParams1D=off  SampleTime=Ts
  Constant8 : Constant  VectorParams1D=off  SampleTime=Ts
  Demux : Demux
  Demux2 : Demux  Outputs=3
  Derivative : Derivative  CoefficientInTFapproximation=Ts
  Display : Display
  Display1 : Display
  Divide : Product  Inputs=*/
  Divide2 : Product  Inputs=***
  Divide3 : Product  Inputs=**
  Logical Operator1 : Logic  AllPortsSameDT=off  OutDataTypeStr=boolean
  Logical Operator5 : Logic  AllPortsSameDT=off  OutDataTypeStr=boolean
  Logical Operator6 : Logic  AllPortsSameDT=off  OutDataTypeStr=boolean
  Math Function : Math  SaturateOnIntegerOverflow=on
  Multiport Switch1 : MultiPortSwitch  Inputs=4
  Multiport Switch2 : MultiPortSwitch  Inputs=4
  Mux : Mux  Inputs=2
  Mux1 : Mux  Inputs=2
  Pickup1 : Constant  Value=[0.1 1 0.6]
  Pickup2 : Constant  Value=Constant_stages
  Product : Product
  Product1 : Product
  Product2 : Product
  Product6 : Product  Inputs=3
  Random Number : RandomNumber  Mean=2  Variance=0.5  SampleTime=Ts
  Scope{1..4,9..10} (6 alike) : Scope
  Switch : Switch  Criteria=u2 > Threshold  InputSameDT=on
  Switch1 : Switch  InputSameDT=on
  Vat : Constant  Value=Vat  SampleTime=Ts
  counter1 : Subsystem
  counter2 : Subsystem
  "m " : Constant  Value=m_Vat  SampleTime=Ts
  Varc : Outport
  TtT_Vp : Outport  Port=2
  TtT_Cid : Outport  Port=3
  tag scope: TIEMPO=global
  wires:
  Random Number/1 -> Divide2/3
  Add4/1 -> Multiport Switch1/3
  Divide2/1 -> Add4/1
  counter1/1(Counter Melting) -> Divide3/1
  [TtT_Cid] -> Product6/3
  Switch1/1 -> Scope10/1, Divide/1
  Demux2/3 -> Multiport Switch2/4
  Pickup1/1 -> Demux2/1
  Demux2/2 -> Multiport Switch2/3
  Multiport Switch2/1 -> [TtT_stage_V], TtT_Vp/1
  Demux2/1 -> Multiport Switch2/2, Multiport Switch2/5
  Product6/1 -> Scope9/1, Add/1
  Product2/1 -> Product6/2
  [TtT_stage_V] -> Product6/1
  In1/1 -> Ajust_1/1, Ajust_1 1/1, Switch/2
  Add1/1 -> Mux1/2, Divide/2
  Demux/2 -> Divide2/1
  Math Function/1 -> Divide2/2
  Demux/3 -> Divide3/2
  Demux/4 -> Multiport Switch1/4, Add4/2
  Pickup2/1 -> Demux/1
  Divide3/1 -> Math Function/1
  Multiport Switch1/1 -> TtT_Cid/1, [TtT_Cid]
  Demux/1 -> Multiport Switch1/5, Multiport Switch1/2
  Condicion arranque5/1 -> Logical Operator6/2
  Logical Operator6/1 -> Add6/2, Logical Operator5/1
  Condicion arranque1/1 -> Logical Operator6/1, Add6/1
  Logical Operator5/1 -> Logical Operator1/1, Add6/3
  Condicion arranque2/1 -> Logical Operator5/2
  Mux1/1 -> Scope3/1
  "Ajust_1 "/1 -> Product/2
  Ajust_1/1 -> Derivative/1
  Derivative/1 -> Switch1/2
  Add2/1 -> Product2/1
  Vat/1 -> Product2/2
  ADD/1 -> Add2/2
  Product1/1 -> Add2/1
  "m "/1 -> Product1/2
  Band-Limited White Noise/1 -> Product1/1
  Abs/1 -> Add1/2, Mux1/1
  Ajust_1 1/1 -> Abs/1
  Constant1/1 -> Add1/1
  Constant5/1 -> Mux/1
  Mux/1 -> Scope1/1
  Constant2/1 -> Switch1/3
  Constant/1 -> Switch1/1
  Product/1 -> Scope2/1, Varc/1, Mux/2
  Switch/1 -> "Ajust_1 "/1
  Constant3/1 -> Switch/1
  Constant4/1 -> Switch/3
  Add/1 -> Product/1
  Divide/1 -> Add/2
  Constant13/1 -> Condicion arranque3/2
  counter2/1(Counter Tap-to_Tap) -> Condicion arranque5/1, Condicion arranque3/1, Condicion arranque2/1, Condicion arranque1/1, Display1/1
  Logical Operator1/1 -> Add6/4
  Condicion arranque3/1 -> Logical Operator1/2
  Add6/1 -> Multiport Switch1/1, counter1/1(In2), Multiport Switch2/1, Display/1, Scope4/1, [TIEMPO]
  Constant6/1 -> Condicion arranque1/2
  Constant7/1 -> Condicion arranque5/2
  Constant8/1 -> Condicion arranque2/2

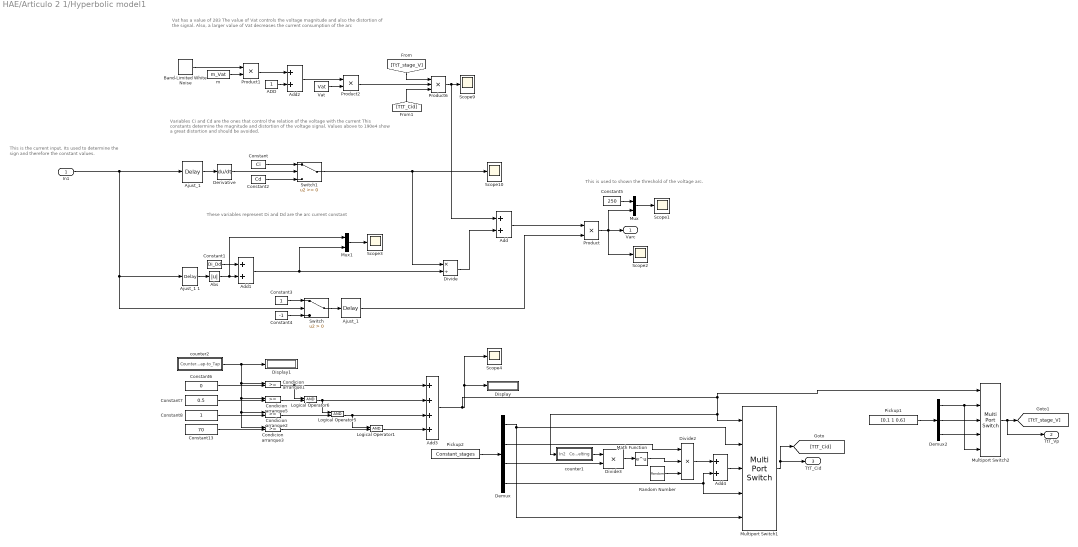
== system HAE/Articulo 2 1/Hyperbolic model1 ==
  note: Vat has a value of 283
      | The value of Vat controls the voltage magnitude and also the distortion of the signal.
      |
      | Also, a larger value of Vat decreases the current consumption of the arc
  note: Variables  Ci and Cd are the ones that control the relation of the voltage with the current
      |
      | This constants determine the magnitude and distortion of the voltage signal.
      |
      | Values above to 190e4 show a great distortion and should be avoided.
  note: These variables represent Di and Dd are the arc current constant
  note: This is used to shown the threshold of the voltage arc.
  note: This is the current input. Its used to determine the sign and therefore the constant values.
  In1 : Inport
  ADD : Constant  SampleTime=Ts
  Abs : Abs
  Add{,1..2,4} (4 alike) : Sum
  Add3 : Sum  Inputs=++++
  Ajust_1 : TransportDelay  DelayTime=1/(1024*60)
  "Ajust_1 " : TransportDelay  DelayTime=1/(1024*60)
  Ajust_1 1 : TransportDelay  DelayTime=1/(1024*60)
  Band-Limited White Noise : simulink/Sources/Band-Limited White Noise  Cov=[0.00005]  Ts=Ts  seed=[500]
  Condicion arranque{1..3,5} (4 alike) : RelationalOperator  OutDataTypeStr=boolean  RndMeth=Nearest
  Constant : Constant  Value=Ci  SampleTime=Ts
  Constant1 : Constant  Value=Di_Dd  SampleTime=Ts
  Constant13 : Constant  Value=70  VectorParams1D=off  SampleTime=Ts
  Constant2 : Constant  Value=Cd
  Constant3 : Constant
  Constant4 : Constant  Value=-1
  Constant5 : Constant  Value=250
  Constant6 : Constant  Value=0  VectorParams1D=off  SampleTime=Ts
  Constant7 : Constant  Value=0.5  VectorParams1D=off  SampleTime=Ts
  Constant8 : Constant  VectorParams1D=off  SampleTime=Ts
  Demux : Demux
  Demux2 : Demux  Outputs=3
  Derivative : Derivative  CoefficientInTFapproximation=Ts
  Display : Display
  Display1 : Display
  Divide : Product  Inputs=*/
  Divide2 : Product  Inputs=***
  Divide3 : Product  Inputs=**
  Logical Operator1 : Logic  AllPortsSameDT=off  OutDataTypeStr=boolean
  Logical Operator5 : Logic  AllPortsSameDT=off  OutDataTypeStr=boolean
  Logical Operator6 : Logic  AllPortsSameDT=off  OutDataTypeStr=boolean
  Math Function : Math  SaturateOnIntegerOverflow=on
  Multiport Switch1 : MultiPortSwitch  Inputs=4
  Multiport Switch2 : MultiPortSwitch  Inputs=4
  Mux : Mux  Inputs=2
  Mux1 : Mux  Inputs=2
  Pickup1 : Constant  Value=[0.1 1 0.6]
  Pickup2 : Constant  Value=Constant_stages
  Product : Product
  Product1 : Product
  Product2 : Product
  Product6 : Product  Inputs=3
  Random Number : RandomNumber  Mean=2  Variance=0.5  SampleTime=Ts
  Scope{1..4,9..10} (6 alike) : Scope
  Switch : Switch  Criteria=u2 > Threshold  InputSameDT=on
  Switch1 : Switch  InputSameDT=on
  Vat : Constant  Value=Vat  SampleTime=Ts
  counter1 : Subsystem
  counter2 : Subsystem
  "m " : Constant  Value=m_Vat  SampleTime=Ts
  Varc : Outport
  TtT_Vp : Outport  Port=2
  TtT_Cid : Outport  Port=3
  wires:
  Random Number/1 -> Divide2/3
  Add4/1 -> Multiport Switch1/3
  Divide2/1 -> Add4/1
  counter1/1(Counter Melting) -> Divide3/1
  [TtT_Cid] -> Product6/3
  Switch1/1 -> Scope10/1, Divide/1
  Demux2/3 -> Multiport Switch2/4
  Pickup1/1 -> Demux2/1
  Demux2/2 -> Multiport Switch2/3
  Multiport Switch2/1 -> [TtT_stage_V], TtT_Vp/1
  Demux2/1 -> Multiport Switch2/2, Multiport Switch2/5
  Product6/1 -> Scope9/1, Add/1
  Product2/1 -> Product6/2
  [TtT_stage_V] -> Product6/1
  In1/1 -> Ajust_1/1, Ajust_1 1/1, Switch/2
  Add1/1 -> Mux1/2, Divide/2
  Demux/2 -> Divide2/1
  Math Function/1 -> Divide2/2
  Demux/3 -> Divide3/2
  Demux/4 -> Multiport Switch1/4, Add4/2
  Pickup2/1 -> Demux/1
  Divide3/1 -> Math Function/1
  Multiport Switch1/1 -> TtT_Cid/1, [TtT_Cid]
  Demux/1 -> Multiport Switch1/5, Multiport Switch1/2
  Mux1/1 -> Scope3/1
  "Ajust_1 "/1 -> Product/2
  Ajust_1/1 -> Derivative/1
  Derivative/1 -> Switch1/2
  Add2/1 -> Product2/1
  Vat/1 -> Product2/2
  ADD/1 -> Add2/2
  Product1/1 -> Add2/1
  "m "/1 -> Product1/2
  Band-Limited White Noise/1 -> Product1/1
  Abs/1 -> Add1/2, Mux1/1
  Ajust_1 1/1 -> Abs/1
  Constant1/1 -> Add1/1
  Constant5/1 -> Mux/1
  Mux/1 -> Scope1/1
  Constant2/1 -> Switch1/3
  Constant/1 -> Switch1/1
  Product/1 -> Scope2/1, Varc/1, Mux/2
  Switch/1 -> "Ajust_1 "/1
  Constant3/1 -> Switch/1
  Constant4/1 -> Switch/3
  Add/1 -> Product/1
  Divide/1 -> Add/2
  Logical Operator1/1 -> Add3/4
  counter2/1(Counter Tap-to_Tap) -> Condicion arranque5/1, Condicion arranque3/1, Condicion arranque2/1, Condicion arranque1/1, Display1/1
  Condicion arranque2/1 -> Logical Operator5/2
  Logical Operator6/1 -> Add3/2, Logical Operator5/1
  Logical Operator5/1 -> Logical Operator1/1, Add3/3
  Condicion arranque3/1 -> Logical Operator1/2
  Condicion arranque1/1 -> Logical Operator6/1, Add3/1
  Condicion arranque5/1 -> Logical Operator6/2
  Add3/1 -> Multiport Switch2/1, counter1/1(In2), Multiport Switch1/1, Scope4/1, Display/1
  Constant13/1 -> Condicion arranque3/2
  Constant6/1 -> Condicion arranque1/2
  Constant7/1 -> Condicion arranque5/2
  Constant8/1 -> Condicion arranque2/2
